simulink model "UAVs_Simulink"  (R2024a)
settings: Solver=FixedStepAuto  StartTime=0.0  StopTime=70  FixedStep=0.01  RelTol=1e-3
values from neighbouring files (symbols this model uses):
  A = [0 1 0 0 0 0 0 0 0 0 0 0 ... (first row only)    [ControlConstants.m]
  B = [0 0 0 0 ... (first row only)    [ControlConstants.m]
  C = [1 0 0 0 0 0 0 0 0 0 0 0 ... (first row only)    [ControlConstants.m]
  K = place(A,B,P)    [ControlConstants.m]
  k_bar = pinv(C*k_bar*B)    [ControlConstants.m]
libraries: simulink x1
settings Model: Creator=joemi  LastModifiedBy=joemi
settings DataIOCC: SaveOutput=off  SignalLogging=off  DSMLogging=off  SaveTime=off  ReturnWorkspaceOutputs=off

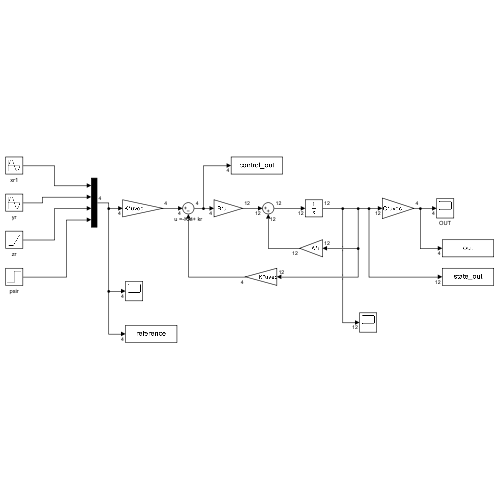
[thumbnail: Simulink's stored preview of the top-level diagram]
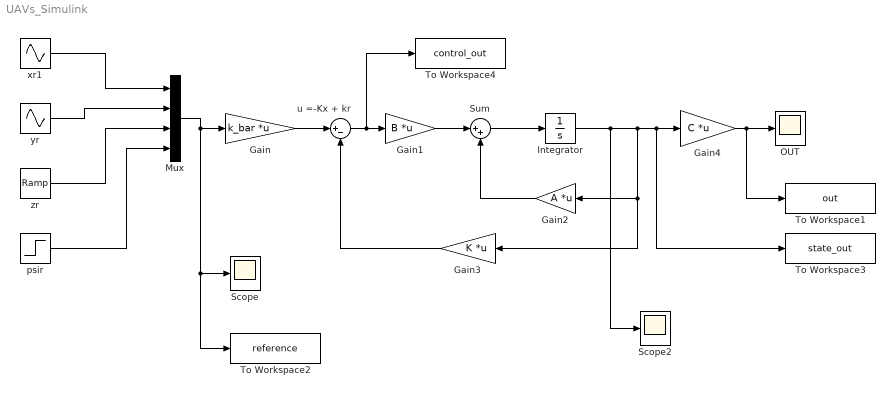
== system UAVs_Simulink ==
  Gain : Gain  Gain=k_bar  Multiplication=Matrix(K*u) (u vector)
  Gain1 : Gain  Gain=B  Multiplication=Matrix(K*u)
  Gain2 : Gain  Gain=A  Multiplication=Matrix(K*u)
  Gain3 : Gain  Gain=K  Multiplication=Matrix(K*u) (u vector)
  Gain4 : Gain  Gain=C  Multiplication=Matrix(K*u) (u vector)
  Integrator : Integrator
  Mux : Mux
  OUT : Scope
  Scope : Scope
  Scope2 : Scope
  Sum : Sum  Inputs=|++
  To Workspace1 : ToWorkspace  VariableName=out  SaveFormat=Timeseries  SampleTime=-1
  To Workspace2 : ToWorkspace  VariableName=reference  SaveFormat=Timeseries  SampleTime=-1
  To Workspace3 : ToWorkspace  VariableName=state_out  SaveFormat=Timeseries  SampleTime=-1
  To Workspace4 : ToWorkspace  VariableName=control_out  SaveFormat=Timeseries  SampleTime=-1
  psir : Step  Time=0  After=0  SampleTime=0
  u =-Kx + kr : Sum  Inputs=|+-
  xr1 : Sin  Amplitude=3  Frequency=0.2  Phase=pi/2  SampleTime=0
  yr : Sin  Amplitude=2  Frequency=0.2  SampleTime=0
  zr : simulink/Sources/Ramp  slope=0.2  start=0  InitialOutput=0
  wires:
  xr1/1 -> Mux/1
  yr/1 -> Mux/2
  zr/1 -> Mux/3
  psir/1 -> Mux/4
  Mux/1 -> Gain/1, To Workspace2/1, Scope/1
  Gain/1 -> u =-Kx + kr/1
  Gain1/1 -> Sum/1
  Sum/1 -> Integrator/1
  Integrator/1 -> Gain4/1, To Workspace3/1, Gain3/1, Gain2/1, Scope2/1
  Gain2/1 -> Sum/2
  Gain3/1 -> u =-Kx + kr/2
  Gain4/1 -> To Workspace1/1, OUT/1
  u =-Kx + kr/1 -> To Workspace4/1, Gain1/1
